simulink model "LimiteCouple"  (R2018a)
settings: Solver=VariableStepAuto  StartTime=0.0  StopTime=250/3.6  RelTol=1e-3
values from neighbouring files (symbols this model uses):
  nr = 0.9    [CaracteristiquesVehicule.m]    (also in UntitFSDAFled.m; getGraphSpeedTorque.m)
  r = 9.73    [CaracteristiquesVehicule.m]    (also in UntitFSDAFled.m; getGraphSpeedTorque.m)
  rr = 0.32995    [CaracteristiquesVehicule.m]    (also in UntitFSDAFled.m = 0.33; getGraphSpeedTorque.m = 0.33)
undefined symbols (not defined in the file or in its folder): Mmax, Pmax, Vmax, Vmin
libraries: simulink x1
settings Model: Creator=thomas.moser  LastModifiedBy=thomas.moser

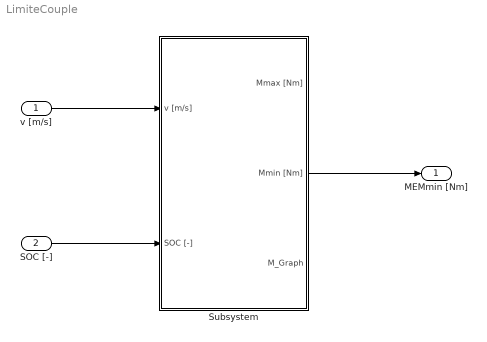
== system LimiteCouple ==
  v [m/s] : Inport
  SOC [-] : Inport  Port=2
  Subsystem : Subsystem
  MEMmin [Nm] : Outport
  wires:
  v [m/s]/1 -> Subsystem/1(v [m/s])
  SOC [-]/1 -> Subsystem/2(SOC [-])
  Subsystem/2(Mmin [Nm]) -> MEMmin [Nm]/1

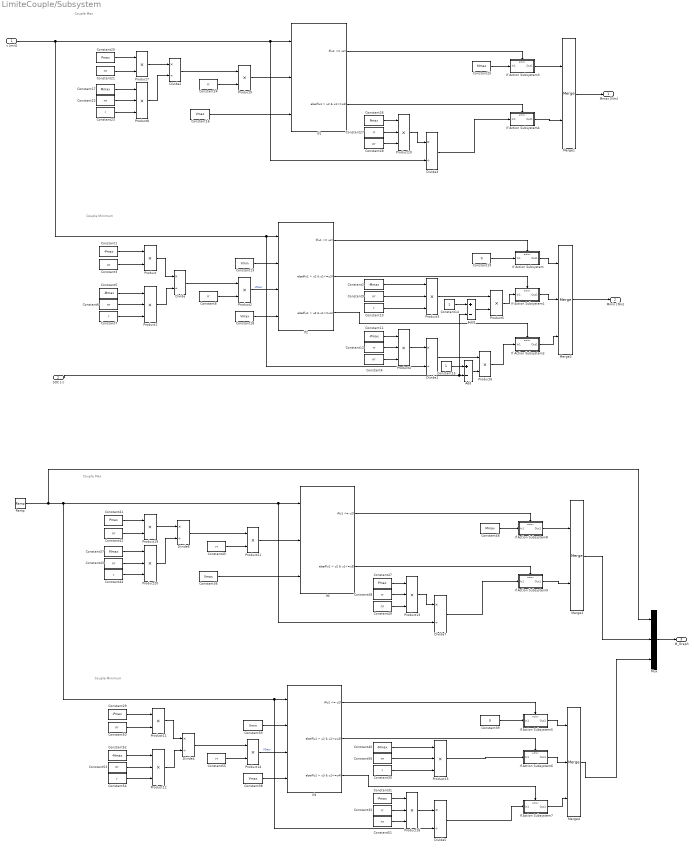
== system LimiteCouple/Subsystem ==
  note: Couple Minimum
  note: Couple Max
  note: Couple Minimum
  note: Couple Max
  v [m/s] : Inport
  SOC [-] : Inport  Port=2
  Add : Sum  Inputs=+-
  Add1 : Sum  Inputs=+-
  Constant{1,11,29,31} (4 alike) : Constant  Value=-Pmax
  Constant{7,10,23,30,44,54} (6 alike) : Constant  Value=r
  Constant{8,12,24,27,32,45,48,55} (8 alike) : Constant  Value=rr
  Constant13 : Constant  Value=Vmin
  Constant14 : Constant
  Constant15 : Constant
  Constant{16,18,36,38} (4 alike) : Constant  Value=Vmax
  Constant{17,25,37,46} (4 alike) : Constant  Value=Mmax
  Constant19 : Constant  Value=0
  Constant{2,5,40,52} (4 alike) : Constant  Value=-Mmax
  Constant{20,26,41,47} (4 alike) : Constant  Value=Pmax
  Constant{3..4,6,9,21..22,28,42..43,49..51,53,56} (14 alike) : Constant  Value=nr
  Constant33 : Constant  Value=Vmin
  Constant39 : Constant  Value=0
  Divide{,1..7} (8 alike) : Product  Inputs=*/
  If Action Subsystem : Subsystem  TreatAsAtomicUnit=on
  If Action Subsystem1 : Subsystem  TreatAsAtomicUnit=on
  If Action Subsystem2 : Subsystem  TreatAsAtomicUnit=on
  If Action Subsystem3 : Subsystem  TreatAsAtomicUnit=on
  If Action Subsystem4 : Subsystem  TreatAsAtomicUnit=on
  If Action Subsystem5 : Subsystem  TreatAsAtomicUnit=on
  If Action Subsystem6 : Subsystem  TreatAsAtomicUnit=on
  If Action Subsystem7 : Subsystem  TreatAsAtomicUnit=on
  If Action Subsystem8 : Subsystem  TreatAsAtomicUnit=on
  If Action Subsystem9 : Subsystem  TreatAsAtomicUnit=on
  If1 : If  NumInputs=3  IfExpression=u1 <= u2  ElseIfExpressions=u1 > u2 & u1<=u3  ShowElse=off
  If2 : If  NumInputs=4  IfExpression=u1 <= u2  ElseIfExpressions=u1 > u2 & u1<=u3, u1 > u3 & u1<=u4  ShowElse=off
  If3 : If  NumInputs=3  IfExpression=u1 <= u2  ElseIfExpressions=u1 > u2 & u1<=u3  ShowElse=off
  If4 : If  NumInputs=4  IfExpression=u1 <= u2  ElseIfExpressions=u1 > u2 & u1<=u3, u1 > u3 & u1<=u4  ShowElse=off
  Merge1 : Merge
  Merge2 : Merge  Inputs=3
  Merge3 : Merge
  Merge4 : Merge  Inputs=3
  Mux : Mux  Inputs=3
  Product{,2,5..7,9,11,14,19,21} (10 alike) : Product
  Product{1,3..4,8,10,12..13,15..16,20} (10 alike) : Product  Inputs=3
  Ramp : simulink/Sources/Ramp  slope=1  start=0  InitialOutput=0
  Mmax [Nm] : Outport
  Mmin [Nm] : Outport  Port=2
  M_Graph : Outport  Port=3
  wires:
  If2/1 -> If Action Subsystem/Action
  Product2/1 -> If2/3  "VDecr"
  Constant4/1 -> Product4/3
  Constant2/1 -> Product3/1
  Product1/1 -> Divide/2
  Constant18/1 -> If2/4
  Product/1 -> Divide/1
  Constant7/1 -> Product1/3
  Add1/1 -> Product5/2
  Constant1/1 -> Product/1
  v [m/s]/1 -> Divide1/2, If2/1, Divide3/2, If1/1
  If2/2 -> If Action Subsystem1/Action
  Divide1/1 -> Product6/1
  Constant3/1 -> Product/2
  Divide/1 -> Product2/1
  Add/1 -> Product6/2
  Constant5/1 -> Product1/1
  Constant6/1 -> Product1/2
  Constant11/1 -> Product4/1
  Constant19/1 -> If Action Subsystem/1(In1)
  Constant9/1 -> Product3/2
  If Action Subsystem/1(Out1) -> Merge2/1
  If Action Subsystem2/1(Out1) -> Merge2/3
  SOC [-]/1 -> Add1/2, Add/2
  Constant13/1 -> If2/2
  Product6/1 -> If Action Subsystem2/1(In1)
  Constant14/1 -> Add1/1
  Product5/1 -> If Action Subsystem1/1(In1)
  If Action Subsystem1/1(Out1) -> Merge2/2
  Merge2/1 -> Mmin [Nm]/1
  If2/3 -> If Action Subsystem2/Action
  Product4/1 -> Divide1/1
  Product3/1 -> Product5/1
  Constant12/1 -> Product4/2
  Constant10/1 -> Product3/3
  Constant8/1 -> Product2/2
  Constant15/1 -> Add/1
  Constant16/1 -> If1/3
  Constant20/1 -> Product7/1
  Constant21/1 -> Product7/2
  Constant17/1 -> Product8/1
  Constant22/1 -> Product8/2
  Constant23/1 -> Product8/3
  Product8/1 -> Divide2/2
  Product7/1 -> Divide2/1
  Divide2/1 -> Product9/1
  Constant24/1 -> Product9/2
  Product9/1 -> If1/2
  If1/1 -> If Action Subsystem3/Action
  Constant25/1 -> If Action Subsystem3/1(In1)
  If Action Subsystem3/1(Out1) -> Merge1/1
  If1/2 -> If Action Subsystem4/Action
  Constant26/1 -> Product10/1
  Constant27/1 -> Product10/2
  Constant28/1 -> Product10/3
  Product10/1 -> Divide3/1
  Divide3/1 -> If Action Subsystem4/1(In1)
  If Action Subsystem4/1(Out1) -> Merge1/2
  Merge1/1 -> Mmax [Nm]/1
  Divide7/1 -> If Action Subsystem9/1(In1)
  If Action Subsystem9/1(Out1) -> Merge3/2
  Product19/1 -> Divide6/1
  If Action Subsystem5/1(Out1) -> Merge4/1
  Constant54/1 -> Product12/3
  Constant56/1 -> Product15/2
  Constant32/1 -> Product16/2
  Product16/1 -> Divide5/1
  If Action Subsystem6/1(Out1) -> Merge4/2
  Constant39/1 -> If Action Subsystem5/1(In1)
  Constant31/1 -> Product16/1
  Constant30/1 -> Product15/3
  Constant55/1 -> Product14/2
  If4/3 -> If Action Subsystem7/Action
  Constant37/1 -> Product20/1
  Constant43/1 -> Product20/2
  Divide6/1 -> Product21/1
  Constant38/1 -> If4/4
  Divide4/1 -> Product14/1
  If4/2 -> If Action Subsystem6/Action
  Constant50/1 -> Product11/2
  If4/1 -> If Action Subsystem5/Action
  Divide5/1 -> If Action Subsystem7/1(In1)
  Product11/1 -> Divide4/1
  Constant36/1 -> If3/3
  Product13/1 -> Divide7/1
  Ramp/1 -> Mux/1, Divide5/2, If4/1, Divide7/2, If3/1
  Constant29/1 -> Product11/1
  Product12/1 -> Divide4/2
  Product14/1 -> If4/3  "VDecr"
  Constant51/1 -> Product16/3
  If Action Subsystem7/1(Out1) -> Merge4/3
  Constant42/1 -> Product19/2
  Product20/1 -> Divide6/2
  Constant53/1 -> Product12/2
  Constant33/1 -> If4/2
  Product21/1 -> If3/2
  Constant52/1 -> Product12/1
  If3/1 -> If Action Subsystem8/Action
  Merge4/1 -> Mux/3
  Constant40/1 -> Product15/1
  Constant47/1 -> Product13/1
  Constant49/1 -> Product13/3
  Constant48/1 -> Product13/2
  Constant41/1 -> Product19/1
  If Action Subsystem8/1(Out1) -> Merge3/1
  Constant46/1 -> If Action Subsystem8/1(In1)
  Constant44/1 -> Product20/3
  Merge3/1 -> Mux/2
  Constant45/1 -> Product21/2
  If3/2 -> If Action Subsystem9/Action
  Product15/1 -> If Action Subsystem6/1(In1)
  Mux/1 -> M_Graph/1

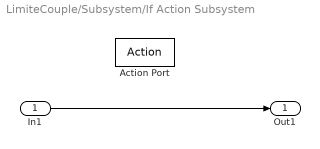
== system LimiteCouple/Subsystem/If Action Subsystem ==
  In1 : Inport
  Action Port : ActionPort  ActionType=then
  Out1 : Outport
  wires:
  In1/1 -> Out1/1

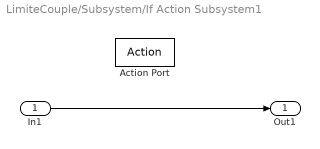
== system LimiteCouple/Subsystem/If Action Subsystem1 ==
  In1 : Inport
  Action Port : ActionPort  ActionType=elseif
  Out1 : Outport
  wires:
  In1/1 -> Out1/1

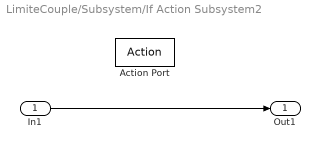
== system LimiteCouple/Subsystem/If Action Subsystem2 ==
  In1 : Inport
  Action Port : ActionPort  ActionType=elseif
  Out1 : Outport
  wires:
  In1/1 -> Out1/1

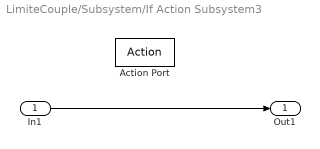
== system LimiteCouple/Subsystem/If Action Subsystem3 ==
  In1 : Inport
  Action Port : ActionPort  ActionType=then
  Out1 : Outport
  wires:
  In1/1 -> Out1/1

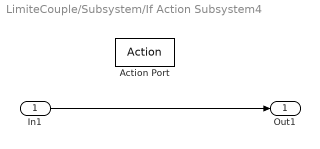
== system LimiteCouple/Subsystem/If Action Subsystem4 ==
  In1 : Inport
  Action Port : ActionPort  ActionType=elseif
  Out1 : Outport
  wires:
  In1/1 -> Out1/1

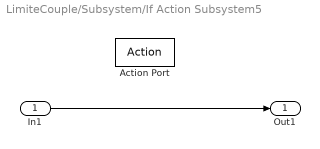
== system LimiteCouple/Subsystem/If Action Subsystem5 ==
  In1 : Inport
  Action Port : ActionPort  ActionType=then
  Out1 : Outport
  wires:
  In1/1 -> Out1/1

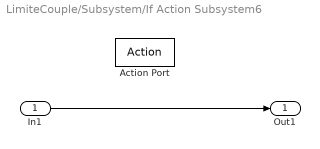
== system LimiteCouple/Subsystem/If Action Subsystem6 ==
  In1 : Inport
  Action Port : ActionPort  ActionType=elseif
  Out1 : Outport
  wires:
  In1/1 -> Out1/1

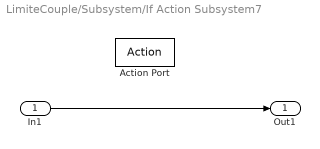
== system LimiteCouple/Subsystem/If Action Subsystem7 ==
  In1 : Inport
  Action Port : ActionPort  ActionType=elseif
  Out1 : Outport
  wires:
  In1/1 -> Out1/1

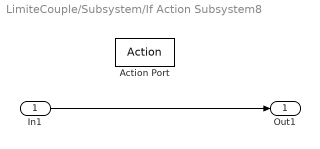
== system LimiteCouple/Subsystem/If Action Subsystem8 ==
  In1 : Inport
  Action Port : ActionPort  ActionType=then
  Out1 : Outport
  wires:
  In1/1 -> Out1/1

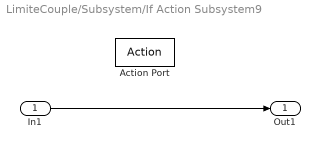
== system LimiteCouple/Subsystem/If Action Subsystem9 ==
  In1 : Inport
  Action Port : ActionPort  ActionType=elseif
  Out1 : Outport
  wires:
  In1/1 -> Out1/1
